simulink model "mmc_model"  (R2025a)
settings: Solver=VariableStepAuto  StartTime=0.0  StopTime=10000  RelTol=1e-3
undefined symbols (not defined in the file): lambda, m, mu, n
settings Model: Creator=Abdullah  LastModifiedBy=Abdullah
settings SolverCC: AlgebraicLoopSolver=TrustRegion
settings DebuggingCC: UnconnectedInputMsg=warning  UnconnectedOutputMsg=warning  UnconnectedLineMsg=warning  ArithmeticOperatorsInVariantConditions=warning
settings ModelReferenceCC: EnableRefExpFcnMdlSchedulingChecks=on
settings SFSimCC: SimUseLocalCustomCode=off  CustomCodeUndefinedFunction=UseInterfaceOnly
settings RTWCC: RTWUseLocalCustomCode=off  GPUComputeCapability=3.5
settings CodeAppCC: StateflowObjectComments=on

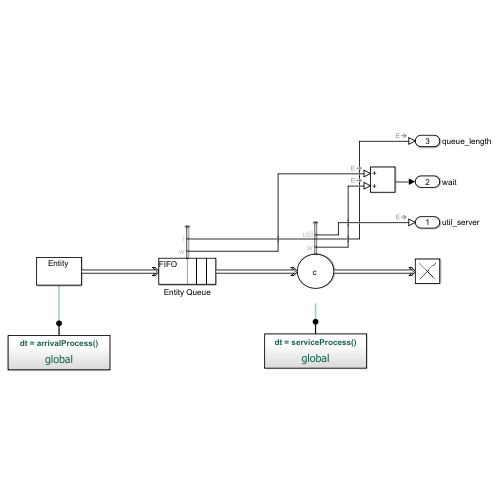
[thumbnail: Simulink's stored preview of the top-level diagram]
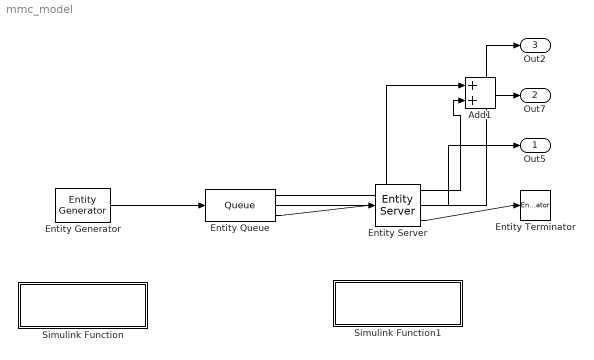
== system mmc_model ==
  Add1 : Sum
  Entity Generator : EntityGenerator  OutputPortMessageModes=m  TimeSource=MATLAB action  IntergenerationTimeAction=dt = arrivalProcess();  EntityType=Structured  EntityTypeName=Entity
  Entity Queue : Queue  InputPortMessageModes=m  OutputPortMessageModes=n,n,m  Capacity=inf  AverageWait=on  AverageQueueLength=on
      settings: OutputPortMap=o2,o3,o5
  Entity Server : EntityServer  InputPortMessageModes=m  OutputPortMessageModes=n,n,m  Capacity=c  ServiceTimeSource=MATLAB action  ServiceTimeAction=dt = serviceProcess();  AverageWait=on  Utilization=on
      settings: OutputPortMap=o4,o5,o9
  Entity Terminator : EntityTerminator  InputPortMessageModes=m
  Simulink Function : Subsystem  TreatAsAtomicUnit=on
  Simulink Function1 : Subsystem  TreatAsAtomicUnit=on
  Out5 : Outport  SignalName=util_server
  Out7 : Outport  Port=2  SignalName=wait
  Out2 : Outport  Port=3  SignalName=queue_length
  wires:
  Entity Generator/1 -> Entity Queue/1
  Entity Queue/3 -> Entity Server/1
  Entity Server/3 -> Entity Terminator/1
  Entity Queue/1 -> Add1/1
  Add1/1 -> Out7/1
  Entity Server/2 -> Out5/1
  Entity Server/1 -> Add1/2
  Entity Queue/2 -> Out2/1

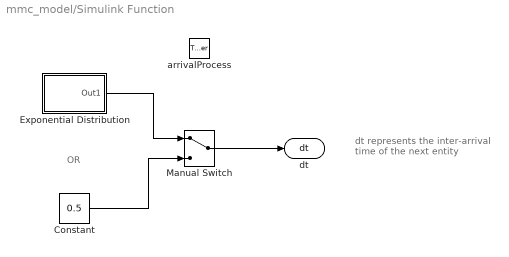
== system mmc_model/Simulink Function ==
  note: OR
  note: dt represents the inter-arrival time of the next entity
  arrivalProcess : TriggerPort  TriggerType=function-call  IsSimulinkFunction=on  FunctionName=arrivalProcess  VariantControl=Variant
  Constant : Constant  Value=0.5
  Exponential Distribution : Subsystem
  Manual Switch : ManualSwitch
  dt : ArgOut  DisableCoverage=on  ArgumentName=dt
  wires:
  Manual Switch/1 -> dt/1
  Exponential Distribution/1(Out1) -> Manual Switch/1
  Constant/1 -> Manual Switch/2

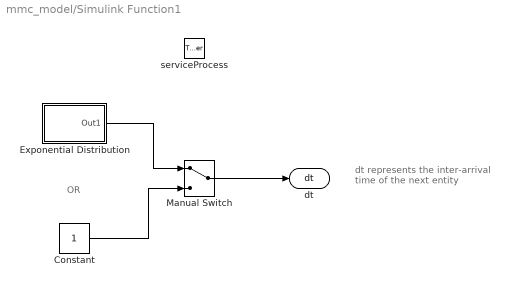
== system mmc_model/Simulink Function1 ==
  note: OR
  note: dt represents the inter-arrival time of the next entity
  serviceProcess : TriggerPort  TriggerType=function-call  IsSimulinkFunction=on  FunctionName=serviceProcess  VariantControl=Variant
  Constant : Constant
  Exponential Distribution : Subsystem
  Manual Switch : ManualSwitch
  dt : ArgOut  DisableCoverage=on  ArgumentName=dt
  wires:
  Manual Switch/1 -> dt/1
  Constant/1 -> Manual Switch/2
  Exponential Distribution/1(Out1) -> Manual Switch/1

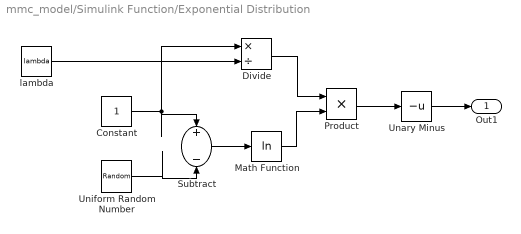
== system mmc_model/Simulink Function/Exponential Distribution ==
  Constant : Constant
  Divide : Product  Inputs=*/
  Math Function : Math  Operator=log
  Product : Product
  Subtract : Sum  Inputs=+-
  Unary Minus : UnaryMinus
  Uniform Random Number : UniformRandomNumber  Minimum=0  Seed=12345
  lambda : Constant  Value=lambda
  Out1 : Outport
  wires:
  Unary Minus/1 -> Out1/1
  lambda/1 -> Divide/2
  Divide/1 -> Product/1
  Subtract/1 -> Math Function/1
  Math Function/1 -> Product/2
  Product/1 -> Unary Minus/1
  Uniform Random Number/1 -> Subtract/2
  Constant/1 -> Divide/1, Subtract/1

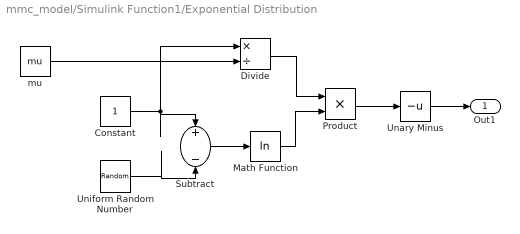
== system mmc_model/Simulink Function1/Exponential Distribution ==
  Constant : Constant
  Divide : Product  Inputs=*/
  Math Function : Math  Operator=log
  Product : Product
  Subtract : Sum  Inputs=+-
  Unary Minus : UnaryMinus
  Uniform Random Number : UniformRandomNumber  Minimum=0  Seed=98765
  mu : Constant  Value=mu
  Out1 : Outport
  wires:
  Unary Minus/1 -> Out1/1
  mu/1 -> Divide/2
  Divide/1 -> Product/1
  Subtract/1 -> Math Function/1
  Math Function/1 -> Product/2
  Product/1 -> Unary Minus/1
  Uniform Random Number/1 -> Subtract/2
  Constant/1 -> Divide/1, Subtract/1
